simulink model "LongitudinalOpenLoop"  (R2020b)
settings: Solver=VariableStepAuto  StartTime=0.0  StopTime=570  RelTol=1e-3
values from neighbouring files (symbols this model uses):
  ALong = [	-0.0141295      0.0580298       0           -9.81 ... (first row only)    [LongitudinalControl.m]
  BLong = [	-0.1703679 ... (first row only)    [LongitudinalControl.m]
  CLong = [1,     0,  0,  0 ... (first row only)    [LongitudinalControl.m]
  DLong = [0 ... (first row only)    [LongitudinalControl.m]
  InitialConditions = [0 ... (first row only)    [LateralControl.m]    (also in LongitudinalControl.m)
settings Model: Creator=Antonis Kantounias  LastModifiedBy=Antonis Kantounias

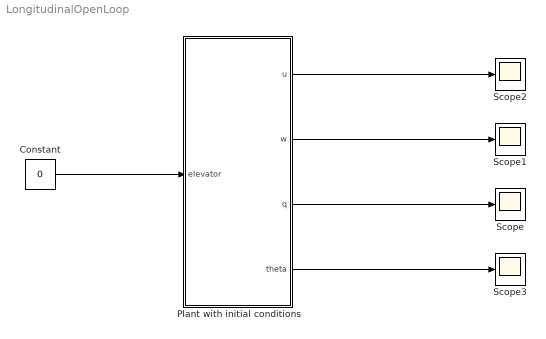
== system LongitudinalOpenLoop ==
  Constant : Constant  Value=0
  Plant with initial conditions : Subsystem
  Scope{,1..3} (4 alike) : Scope
  wires:
  Constant/1 -> Plant with initial conditions/1(elevator)
  Plant with initial conditions/3(q) -> Scope/1
  Plant with initial conditions/1(u) -> Scope2/1
  Plant with initial conditions/2(w) -> Scope1/1
  Plant with initial conditions/4(theta) -> Scope3/1

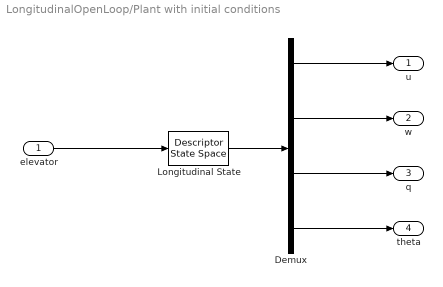
== system LongitudinalOpenLoop/Plant with initial conditions ==
  elevator : Inport
  Demux : Demux
  "Longitudinal State " : DescriptorStateSpace  E=ELong  A=ALong  B=BLong  C=CLong  D=DLong  InitialCondition=InitialConditions  ContinuousStateAttributes='LongitudinalSystem'
  u : Outport
  w : Outport  Port=2
  q : Outport  Port=3
  theta : Outport  Port=4
  wires:
  "Longitudinal State "/1 -> Demux/1
  Demux/4 -> theta/1
  Demux/1 -> u/1
  Demux/3 -> q/1
  Demux/2 -> w/1
  elevator/1 -> "Longitudinal State "/1
